simulink model "Ardunio_SmartHomeMDL"  (R2016a)
settings: Solver=VariableStepAuto  StartTime=0.0  StopTime=10.0  RelTol=1e-3
libraries: arduinolib x5
settings Model: Creator=Mohamed Fawzy  LastModifiedBy=Mohamed Fawzy

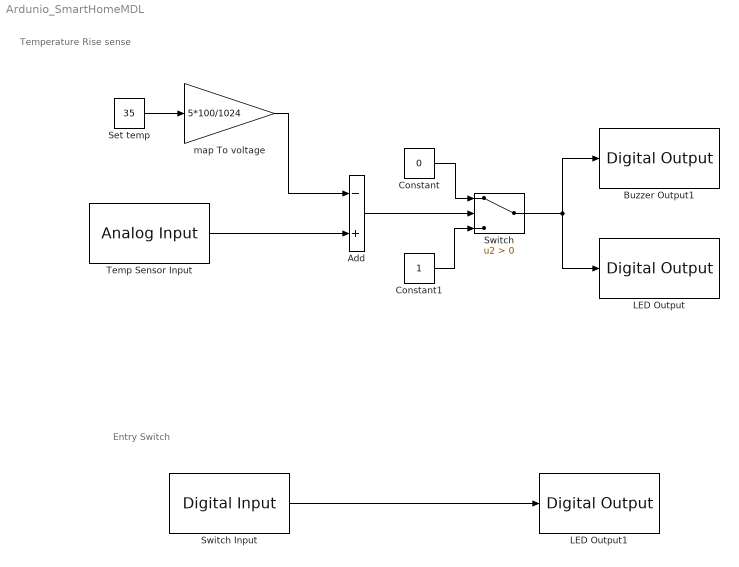
== system Ardunio_SmartHomeMDL ==
  note: Temperature Rise sense
  note: Entry Switch
  Add : Sum  Inputs=-+
  Buzzer Output1 : arduinolib/Digital Output  pinNumber=11  blockPlatform=arduino
  Constant : Constant  Value=0
  Constant1 : Constant
  LED Output : arduinolib/Digital Output  pinNumber=10  blockPlatform=arduino
  LED Output1 : arduinolib/Digital Output  pinNumber=9  blockPlatform=arduino
  "Set temp " : Constant  Value=35
  Switch : Switch  Criteria=u2 > Threshold
  Switch Input : arduinolib/Digital Input  pinNumber=8  sampleTime=1  blockPlatform=arduino
  Temp Sensor Input : arduinolib/Analog Input  pinNumber=4  sampleTime=1  blockPlatform=arduino
  "map To voltage " : Gain  Gain=5*100/1024
  wires:
  Switch Input/1 -> LED Output1/1
  Switch/1 -> LED Output/1, Buzzer Output1/1
  Constant/1 -> Switch/1
  Constant1/1 -> Switch/3
  "Set temp "/1 -> "map To voltage "/1
  Add/1 -> Switch/2
  "map To voltage "/1 -> Add/1
  Temp Sensor Input/1 -> Add/2
